simulink library "libc_extended_basics"  (R2015b)
settings: Solver=FixedStepDiscrete  StartTime=0.0  StopTime=Inf  FixedStep=0.004  RelTol=1e-3
PostLoadFcn:
  | , if any(exist('dsrtsu_mdlpostloadfcn', 'file') == [2, 3, 6]), try dsrtsu_mdlpostloadfcn('Execute', bdroot); catch fprintf('Error in PostLoadFcn (dsrtsu_mdlpostloadfcn) for model "%s":\n %s\n', bdroot, lasterr); end, end,
libraries: simulink x3
settings Model: DSRTSU_INTERNAL_RTI_VER=470  DSRTSU_INTERNAL_RTI_TYPE=rti1007  DSRTSU_INTERNAL_RTIFPGA=60  Creator=Falkenhahn  LastModifiedBy=isysfalkenhahn
settings DataIOCC: SaveFormat=Array
settings OptimizationCC: BlockReduction=off  OptimizeBlockIOStorage=off  BufferReuse=off  GlobalBufferReuse=off  ExpressionFolding=off  LocalBlockOutputs=off
settings DebuggingCC: UnderspecifiedInitializationDetection=Classic  MergeDetectMultiDrivingBlocksExec=none  SolverPrmCheckMsg=warning
settings HardwareCC: ProdBitPerPointer=32  ProdLargestAtomicFloat=None  ProdEndianess=BigEndian  ProdWordSize=32  ProdHWDeviceType=Generic->Custom  TargetIntDivRoundTo=Zero  TargetEndianess=BigEndian  TargetHWDeviceType=Generic->Custom
settings RTWCC: SystemTargetFile=rti1007.tlc  MakeCommand=make_rti  TemplateMakefile=rti1007.tmf  Description=dSPACE DS1007 Hardware Platform
settings STFCustomTargetCC: ParMdlRefBuildCompliant=on  ConcurrentExecutionCompliant=off  MatFileLogging=on  SystemTargetFile=rti1007.tlc
settings GRTTargetCC: CompOptLevelCompliant=off  ConcurrentExecutionCompliant=off  GeneratePreprocessorConditionals=Disable all  CombineOutputUpdateFcns=off  GRTInterface=on  UseToolchainInfoCompliant=off  ExtModeMexFile=noextcomm
settings ConfigComp: CovModelRefEnable=Off

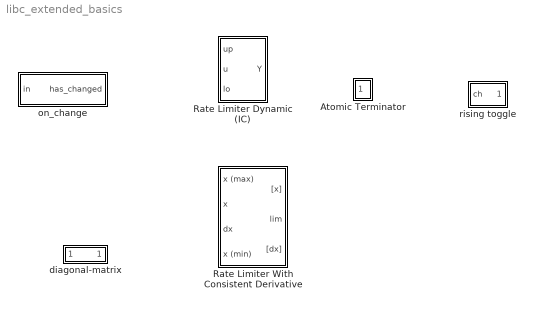
== system libc_extended_basics ==
  Atomic Terminator : Subsystem  TreatAsAtomicUnit=on
  Rate Limiter Dynamic (IC) : Subsystem  mask(Rate Limiter Dynamic (IC)){}
      mask help:
      | Modifizierter Simulink-Block: Der interne Unit-Delay-Block übernimmt die Initial Condition vom Eingang.
      |
      | Limit rising and falling rates of the signals at the second input by using the first input (upper limit) and the third input (lower limit).
      mask Display: plot([0.15 0.95],[.5 .5],[.5 .5],[0.05 0.95],0.05+0.9*[.2 .8],0.05+0.9*[0 1]);
  Rate Limiter With Consistent Derivative : Subsystem
      mask Display: plot([0.15 0.85],[.5 .5],[.5 .5],[0.05 0.95],0.15+0.7*[0 .25 .75 1],0.05+0.9*[.25 .25 .75 .75]);
  diagonal-matrix : Subsystem
  on_change : Subsystem  mask{IC=-1}
      mask prompts: IC "Initial condition"
      mask help: Select the initial condition to be //different// from the initial input to force an initial output at program start.
  rising toggle : Subsystem

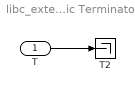
== system libc_extended_basics/Atomic Terminator ==
  T : Inport
  T2 : Terminator
  wires:
  T/1 -> T2/1

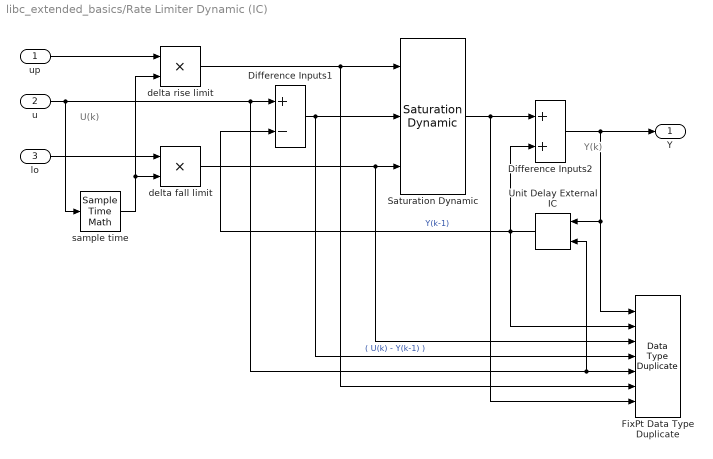
== system libc_extended_basics/Rate Limiter Dynamic (IC) ==
  note: Y(k)
  note: U(k)
  up : Inport
  u : Inport  Port=2
  lo : Inport  Port=3
  Difference Inputs1 : Sum  Description=Add in CPU  DisableCoverage=on  Inputs=+-  OutDataTypeStr=Inherit: Inherit via back propagation
  Difference Inputs2 : Sum  Description=Add in CPU  OutDataTypeStr=Inherit: Inherit via back propagation
  FixPt Data Type Duplicate : DataTypeDuplicate  DisableCoverage=on  NumInputPorts=7
  Saturation Dynamic : simulink/Discontinuities/Saturation Dynamic  OutMin=[]  OutMax=[]  OutDataTypeStr=Inherit: Same as second input  OutDataType=fixdt(1, 16)  OutScaling=2^-10  DoSatur=off
  Unit Delay External IC : simulink/Additional Math & Discrete/Additional Discrete/Unit Delay External IC  tsamp=-1
  delta fall limit : Product  DisableCoverage=on  Inputs=**  OutDataTypeStr=Inherit: Inherit via back propagation  SaturateOnIntegerOverflow=on
  delta rise limit : Product  DisableCoverage=on  Inputs=**  OutDataTypeStr=Inherit: Inherit via back propagation  SaturateOnIntegerOverflow=on
  sample time : SampleTimeMath  DisableCoverage=on  TsampMathOp=Ts Only  weightValue=1
  Y : Outport  InitialOutput=0
  wires:
  Difference Inputs1/1 -> FixPt Data Type Duplicate/4, Saturation Dynamic/2  "( U(k) - Y(k-1) )"
  u/1 -> Difference Inputs1/1, FixPt Data Type Duplicate/5, Unit Delay External IC/2, sample time/1
  delta fall limit/1 -> FixPt Data Type Duplicate/3, Saturation Dynamic/3
  Saturation Dynamic/1 -> Difference Inputs2/1, FixPt Data Type Duplicate/7
  Unit Delay External IC/1 -> Difference Inputs2/2, Difference Inputs1/2, FixPt Data Type Duplicate/2  "Y(k-1)"
  Difference Inputs2/1 -> Y/1, Unit Delay External IC/1, FixPt Data Type Duplicate/1
  up/1 -> delta rise limit/1
  delta rise limit/1 -> FixPt Data Type Duplicate/6, Saturation Dynamic/1
  lo/1 -> delta fall limit/1
  sample time/1 -> delta fall limit/2, delta rise limit/2

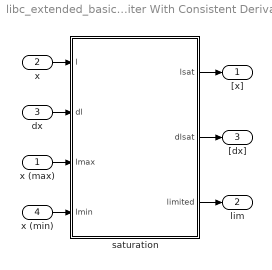
== system libc_extended_basics/Rate Limiter With Consistent Derivative ==
  x (max) : Inport
  x : Inport  Port=2
  dx : Inport  Port=3
  x (min) : Inport  Port=4
  saturation : MATLAB Function  TreatAsAtomicUnit=on
  "[x]" : Outport
  lim : Outport  Port=2
  "[dx]" : Outport  Port=3
  wires:
  x (max)/1 -> saturation/3(lmax)
  dx/1 -> saturation/2(dl)
  x/1 -> saturation/1(l)
  saturation/2(dlsat) -> "[dx]"/1
  saturation/1(lsat) -> "[x]"/1
  x (min)/1 -> saturation/4(lmin)
  saturation/3(limited) -> lim/1

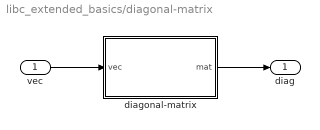
== system libc_extended_basics/diagonal-matrix ==
  vec : Inport
  diagonal-matrix : MATLAB Function  TreatAsAtomicUnit=on
  diag : Outport
  wires:
  vec/1 -> diagonal-matrix/1(vec)
  diagonal-matrix/1(mat) -> diag/1

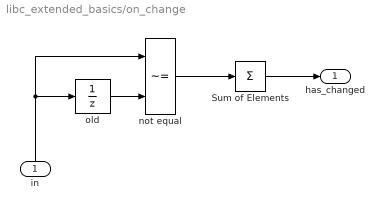
== system libc_extended_basics/on_change ==
  in : Inport
  Sum of Elements : Sum  Inputs=+
  not equal : RelationalOperator  Operator=~=  OutDataTypeStr=boolean
  old : UnitDelay  InitialCondition=IC  SampleTime=-1
  has_changed : Outport
  wires:
  Sum of Elements/1 -> has_changed/1
  in/1 -> not equal/1, old/1
  old/1 -> not equal/2
  not equal/1 -> Sum of Elements/1

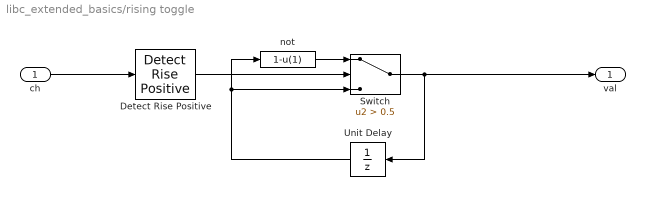
== system libc_extended_basics/rising toggle ==
  ch : Inport
  Detect Rise Positive : simulink/Logic and Bit Operations/Detect Rise Positive  vinit=0  InputProcessing=Inherited  OutDataTypeStr=boolean
  Switch : Switch  Criteria=u2 > Threshold  Threshold=0.5
  Unit Delay : UnitDelay  SampleTime=-1
  not : Fcn  Expr=1-u(1)
  val : Outport
  wires:
  Detect Rise Positive/1 -> Switch/2
  Switch/1 -> val/1, Unit Delay/1
  ch/1 -> Detect Rise Positive/1
  not/1 -> Switch/1
  Unit Delay/1 -> Switch/3, not/1

== matlab function libc_extended_basics/diagonal-matrix/diagonal-matrix ==
  data: vec input; mat output
function mat = diag(vec)

mat = diag(vec);

== matlab function libc_extended_basics/Rate Limiter With Consistent Derivative/saturation ==
  data: l input; lsat output; dlsat output; limited output; dl input; lmax input; lmin input
function [lsat, dlsat, limited] = saturation(l, dl, lmax, lmin)
%#codegen

lsat = min(max(l,lmin),lmax);
dlsat = dl;

% Identifizieren, wo Limits sind
limited = ((lsat - l) < 0) - ((lsat - l) > 0);

% Begrenze Geschwindigkeit zu 0, wo die Länge nach oben bzw. nach unten
% beschränkt wurde.
dlsat = min(dlsat, ((lsat - l) >= 0).*dlsat); % Obere Schranke
dlsat = max(dlsat, ((lsat - l) <= 0).*dlsat); % Untere Schranke
